simulink model "ICdesign_intro"  (R2017a)
settings: Solver=VariableStepAuto  StartTime=0.0  StopTime=10  RelTol=1e-3
libraries: dspsrcs4 x2, dspfdesign x1
settings Model: Creator=Arthur  LastModifiedBy=Arthur

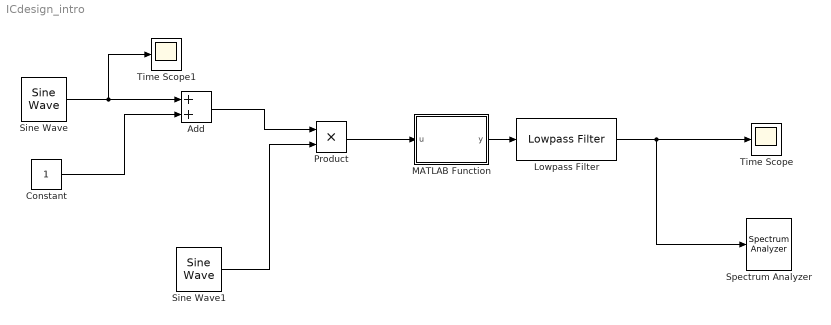
== system ICdesign_intro ==
  Add : Sum
  Constant : Constant
  Lowpass Filter : dspfdesign/Lowpass Filter  FilterType=FIR  DesignForMinimumOrder=on  FilterOrder=50  PassbandFrequency=500  StopbandFrequency=800  PassbandRipple=1  StopbandAttenuation=30  InheritSampleRate=off  SampleRate=4000  SimulateUsing=Interpreted execution  roundingMode=Floor  coeffsDataTypeStr=fixdt(1,16)
  MATLAB Function : MATLAB Function  TreatAsAtomicUnit=on
  Product : Product
  Sine Wave : dspsrcs4/Sine Wave  Amplitude=1  Frequency=5  Phase=0  SampleMode=Discrete  OutComplex=Real  CompMethod=Trigonometric fcn  TableSize=Speed  SampleTime=1/1000  SamplesPerFrame=1  ResetState=Restart at time zero  OutputFrames=off  dataType=double  wordLen=16  udDataType=sfix(16)  fracBitsMode=Best precision  numFracBits=15  OutDataTypeStr=double  LastOutDataTypeStr=double
  Sine Wave1 : dspsrcs4/Sine Wave  Amplitude=1  Frequency=500  Phase=0  SampleMode=Discrete  OutComplex=Real  CompMethod=Trigonometric fcn  TableSize=Speed  SampleTime=1/1000  SamplesPerFrame=1  ResetState=Restart at time zero  OutputFrames=off  dataType=double  wordLen=16  udDataType=sfix(16)  fracBitsMode=Best precision  numFracBits=15  OutDataTypeStr=double  LastOutDataTypeStr=double
  Spectrum Analyzer : SpectrumAnalyzer
  Time Scope : Scope
  Time Scope1 : Scope
  wires:
  Constant/1 -> Add/2
  Sine Wave/1 -> Time Scope1/1, Add/1
  Add/1 -> Product/1
  Sine Wave1/1 -> Product/2
  Product/1 -> MATLAB Function/1(u)
  MATLAB Function/1(y) -> Lowpass Filter/1
  Lowpass Filter/1 -> Spectrum Analyzer/1, Time Scope/1

== matlab function ICdesign_intro/MATLAB Function ==
  data: u input; y output
function y = fcn(u)

y = abs(u);
